simulink model "generator_of_pseudo_measures"  (R2016b)
settings: Solver=ode8  StartTime=0.0  StopTime=50  FixedStep=0.1  RelTol=1e-3
undefined symbols (not defined in the file or in its folder): deg, rad, s
libraries: simulink x6, powerlib_meascontrol x3, dspsrcs4 x3, aerolibconvert2 x2, aerolib6dof2 x1
settings Model: Creator=Utente  LastModifiedBy=liana

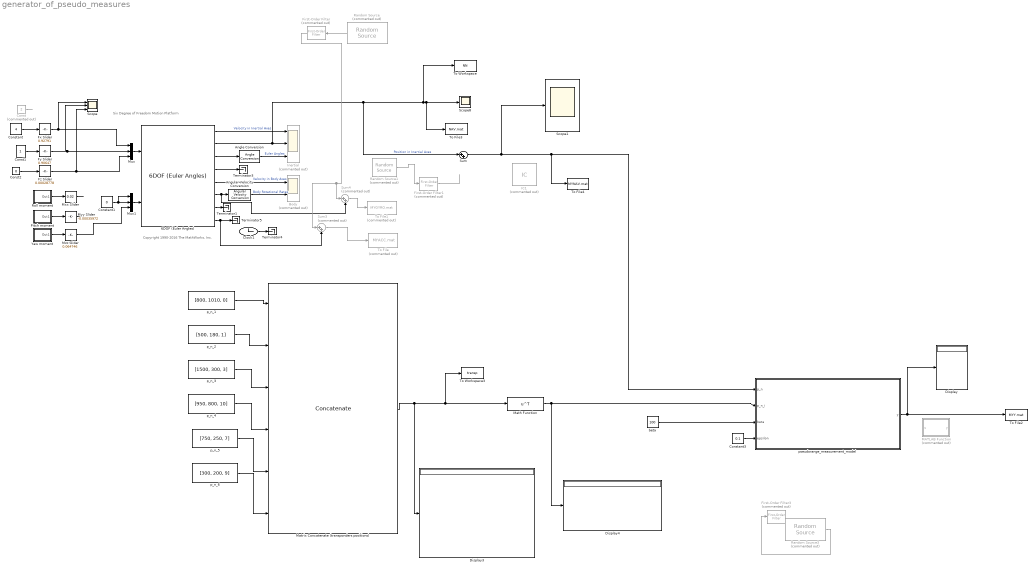
== system generator_of_pseudo_measures ==
  note: Six Degree of Freedom Motion Platform
  note: Copyright 1990-2016 The MathWorks, Inc.
  6DOF (Euler Angles) : aerolib6dof2/6DOF (Euler Angles)  units=Metric (MKS)  mtype=Fixed  rep=Euler Angles  xme_0=[0 0 0]  Vm_0=[0 0 0]  eul_0=[0 0 0]  pm_0=[0 0 0]  mass_0=1.0  mass_e=0.5  mass_f=2.0  inertia=eye(3)  inertia_e=eye(3)  inertia_f=2*eye(3)  k_quat=1.0  vre_flag=on
  Angle Conversion : aerolibconvert2/Angle Conversion  IU=rad  OU=deg
  Angular Velocity Conversion : aerolibconvert2/Angular Velocity Conversion  IU=rad/s  OU=deg/s
  Body : Scope  Commented=on  NumInputPorts=2
  Clock1 : Clock
      settings: Decimation=100
  Const : Constant  Commented=on  Value=2
  Const1 : Constant
  Const2 : Constant  Value=0
  Constant : Constant  Value=4
  Constant1 : Constant  Value=0
  Constant3 : Constant  Value=0.1
  Display : Display
  Display3 : Display
  Display4 : Display
  First-Order Filter : powerlib_meascontrol/Filters/First-Order Filter  Commented=on  FilterType=Lowpass  Tc=10  Ts=0  Initialize=on  Vac_Init=[0, 0, 60]  Vdc_Init=0  PlotResponse=off  FreqRange="[0,  200,  1]"
  First-Order Filter1 : powerlib_meascontrol/Filters/First-Order Filter  Commented=on  FilterType=Lowpass  Tc=100  Ts=0.1  Initialize=on  Vac_Init=[0, 0, 0]  Vdc_Init=0  PlotResponse=off  FreqRange="[0,  200,  1]"
  First-Order Filter3 : powerlib_meascontrol/Filters/First-Order Filter  Commented=on  FilterType=Lowpass  Tc=10  Ts=0  Initialize=on  Vac_Init=[0, 0, 60]  Vdc_Init=0  PlotResponse=off  FreqRange="[0,  200,  1]"
  Fx Slider : simulink/Math Operations/Slider Gain  low=-1  gain=0.92791  high=1
  Fy Slider : simulink/Math Operations/Slider Gain  low=-1  gain=0.90647  high=1
  Fz Slider : simulink/Math Operations/Slider Gain  low=-1  gain=0.00028778  high=1
  IC1 : InitialCondition  Commented=on  Value=[100;100;100]
  Inertial : Scope  Commented=on  NumInputPorts=3
  MATLAB Function : MATLAB Function  Commented=on  TreatAsAtomicUnit=on
  Math Function : Math  Operator=transpose  SaturateOnIntegerOverflow=on
  Matrix Concatenate (transponders positions) : Concatenate  NumInputs=6  Mode=Multidimensional array  ConcatenateDimension=2
  Mux : Mux  Inputs=3
  Mux1 : Mux  Inputs=3
  Mxx Slider : simulink/Math Operations/Slider Gain  low=0  gain=0.02  high=1
  Myy Slider : simulink/Math Operations/Slider Gain  low=-5  gain=-0.00035972  high=1
  Mzz Slider : simulink/Math Operations/Slider Gain  low=-3  gain=0.064746  high=3
  Pitch moment : Subsystem  mask(timed input){t=[0 3 3 4 4 5 5  7.5 7.5 8.5 8.5 9.5 9.5 10], u=[0 0  1 1 -1 -1.005 0 0 -1 -1 1 1 0 0]*3.138/2}
      mask prompts: t "time values:"; u "input values"
      mask Display: plot(t,u)
  Random Source : dspsrcs4/Random Source  Commented=on  SrcType=Gaussian  NormMethod=Ziggurat  CltLength=12  MinVal=0  MaxVal=1  MeanVal=[0;0;0]  VarVal=[1;1;1]  RepMode=Repeatable  rawSeed=1  IsInherit=off  SampMode=Continuous  SampTime=0.1  SampFrame=1  DataType=Double  OutComplex=Real  OutputFrames=off
  Random Source1 : dspsrcs4/Random Source  Commented=on  SrcType=Gaussian  NormMethod=Ziggurat  CltLength=12  MinVal=0  MaxVal=1  MeanVal=[0;0;0]  VarVal=[1;1;1]*100  RepMode=Not repeatable  rawSeed=1  IsInherit=off  SampMode=Discrete  SampTime=0.1  SampFrame=1  DataType=Double  OutComplex=Real  OutputFrames=off
  Random Source3 : dspsrcs4/Random Source  Commented=on  SrcType=Gaussian  NormMethod=Ziggurat  CltLength=12  MinVal=0  MaxVal=1  MeanVal=0.5  VarVal=0.1  RepMode=Repeatable  rawSeed=1  IsInherit=off  SampMode=Continuous  SampTime=0.1  SampFrame=1  DataType=Double  OutComplex=Real  OutputFrames=off
  Roll moment : Subsystem  mask(timed input){t=[0 1 1 2 2  10], u=[1 1 -1 -.998  0 0]*3.144/2}
      mask prompts: t "time values:"; u "input values"
      mask Display: plot(t,u)
  Scope : Scope  NumInputPorts=3
  Scope1 : Scope
  Scope8 : Scope
  Sum : Sum  Inputs=|++
  Sum3 : Sum  Commented=on  Inputs=|++
  Sum4 : Sum  Commented=on  Inputs=|++
  Terminator{1,3..5} (4 alike) : Terminator
  To File : ToFile  Commented=on  Filename=MYACC.mat  SaveFormat=Timeseries
  To File1 : ToFile  Commented=on  Filename=MYGYRO.mat  SaveFormat=Timeseries
  To File2 : ToFile  Filename=MYY.mat  SaveFormat=Timeseries
  To File3 : ToFile  Filename=NAV.mat  SaveFormat=Timeseries
  To File4 : ToFile  Filename=MYNAV.mat  SaveFormat=Timeseries
  To Workspace : ToWorkspace  VariableName=NN  SaveFormat=Timeseries  SampleTime=-1
  To Workspace3 : ToWorkspace  VariableName=transp  SaveFormat=Timeseries  SampleTime=-1
  Yaw moment : Subsystem  mask(timed input){t=[0 2 4 6 8 10], u=[0 1  1 1 -1 0]*3.1/2}
      mask prompts: t "time values:"; u "input values"
      mask Display: plot(t,u)
  beta : Constant  Value=100
  p_n_1 : Constant  Value=[800, 1010, 0]
  p_n_2 : Constant  Value=[500, 180, 1]
  p_n_3 : Constant  Value=[1500, 300, 3]
  p_n_4 : Constant  Value=[950, 800, 10]
  p_n_5 : Constant  Value=[750, 250, 7]
  p_n_6 : Constant  Value=[300, 200, 9]
  pseudorange_measurement_model : MATLAB Function  TreatAsAtomicUnit=on
  wires:
  Yaw moment/1(Out1) -> Mzz Slider/1
  Pitch moment/1(Out1) -> Myy Slider/1
  Roll moment/1(Out1) -> Mxx Slider/1
  Const2/1 -> Fz Slider/1
  Const1/1 -> Fy Slider/1
  Clock1/1 -> Terminator4/1
  Mux1/1 -> 6DOF (Euler Angles)/2
  Mzz Slider/1 -> Mux1/3
  Myy Slider/1 -> ?
  Mxx Slider/1 -> ?
  Mux/1 -> 6DOF (Euler Angles)/1
  Fy Slider/1 -> Scope/2, Mux/2
  Fz Slider/1 -> Scope/3, Mux/3
  Fx Slider/1 -> Mux/1, Scope/1
  6DOF (Euler Angles)/4 -> Terminator3/1
  6DOF (Euler Angles)/7 -> Terminator1/1
  6DOF (Euler Angles)/3 -> Angle Conversion/1
  6DOF (Euler Angles)/5 -> Body/1  "Velocity in Body Axes"
  6DOF (Euler Angles)/1 -> Inertial/1  "Velocity in Inertial Axes"
  6DOF (Euler Angles)/2 -> Sum/1, To Workspace/1, To File3/1, Scope8/1, Inertial/2  "Position in Inertial Axes"
  Angle Conversion/1 -> Inertial/3  "Euler Angles"
  6DOF (Euler Angles)/6 -> Sum4/2, Angular Velocity Conversion/1
  Angular Velocity Conversion/1 -> Body/2  "Body Rotational Rates"
  6DOF (Euler Angles)/8 -> Sum3/2, Terminator5/1
  Random Source/1 -> First-Order Filter/1
  First-Order Filter/1 -> Sum3/1, Sum4/1
  Const/1 -> ?
  Constant1/1 -> Mux1/1, Mux1/2
  Sum3/1 -> To File/1
  Sum4/1 -> To File1/1
  Matrix Concatenate (transponders positions)/1 -> To Workspace3/1, Math Function/1, Display3/1
  Math Function/1 -> Display4/1, pseudorange_measurement_model/2(p_n_i)
  p_n_1/1 -> Matrix Concatenate (transponders positions)/1
  p_n_2/1 -> Matrix Concatenate (transponders positions)/2
  p_n_3/1 -> Matrix Concatenate (transponders positions)/3
  p_n_4/1 -> Matrix Concatenate (transponders positions)/4
  p_n_5/1 -> Matrix Concatenate (transponders positions)/5
  Random Source3/1 -> First-Order Filter3/1
  Constant3/1 -> pseudorange_measurement_model/4(epsilon)
  beta/1 -> pseudorange_measurement_model/3(beta)
  p_n_6/1 -> Matrix Concatenate (transponders positions)/6
  Random Source1/1 -> First-Order Filter1/1
  pseudorange_measurement_model/1(y) -> Display/1, To File2/1
  First-Order Filter1/1 -> ?
  Sum/1 -> Scope1/1, pseudorange_measurement_model/1(p_n), To File4/1
  Constant/1 -> Fx Slider/1

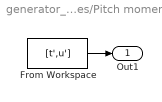
== system generator_of_pseudo_measures/Pitch moment ==
  From Workspace : FromWorkspace  VariableName=[t',u']  SampleTime=0
  Out1 : Outport
  wires:
  From Workspace/1 -> Out1/1

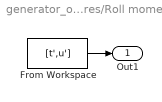
== system generator_of_pseudo_measures/Roll moment ==
  From Workspace : FromWorkspace  VariableName=[t',u']  SampleTime=0
  Out1 : Outport
  wires:
  From Workspace/1 -> Out1/1

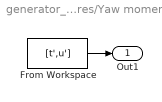
== system generator_of_pseudo_measures/Yaw moment ==
  From Workspace : FromWorkspace  VariableName=[t',u']  SampleTime=0
  Out1 : Outport
  wires:
  From Workspace/1 -> Out1/1

== matlab function generator_of_pseudo_measures/MATLAB Function ==
  data: u input; y output
function y = fcn(u)

y = zeros(6,1);

y = u;

y(4,1) = 0;

== matlab function generator_of_pseudo_measures/pseudorange_measurement_model ==
  data: p_n input; y output size=[6,1]; p_n_i input; beta input; epsilon input
function y = pseudorange_mea_model(p_n, p_n_i, beta, epsilon)

  %  row-vector
  
  [r,c] = size(p_n_i);
  
  p_n_i = p_n_i';

  y = zeros(r,1);

  for i=1:1:r

%       rho = norm(p_n - (p_n_i(i,:))');  % eq. 7
      rho = norm(p_n - p_n_i(:,i),2);  
      
      y(i) = rho + beta + epsilon; % eq. 8 

  end
      
end
